simulink model "cyclo_mt"  (R2015b)
settings: Solver=FixedStepAuto  StartTime=0.0  StopTime=0.05  RelTol=1e-3
PreLoadFcn:
  | Ts=1e-6;
InitFcn:
  | DeadZone = 5;
  | block_angle = 90 - DeadZone;
  | Ts  = 1e-6;
  | fref = 50;
  | Eref = 400;
  | Em  = 4.16e3 * sqrt(2) / sqrt(3);
  | fao = 0;
undefined symbols (not defined in the file): D1, Delta, DiscIntNeverNeededParam, lagging, pulse
libraries: powerlib x26, powerlib_meascontrol x15, simulink x8
settings Model: Creator=fujitsu  LastModifiedBy=fujitsu

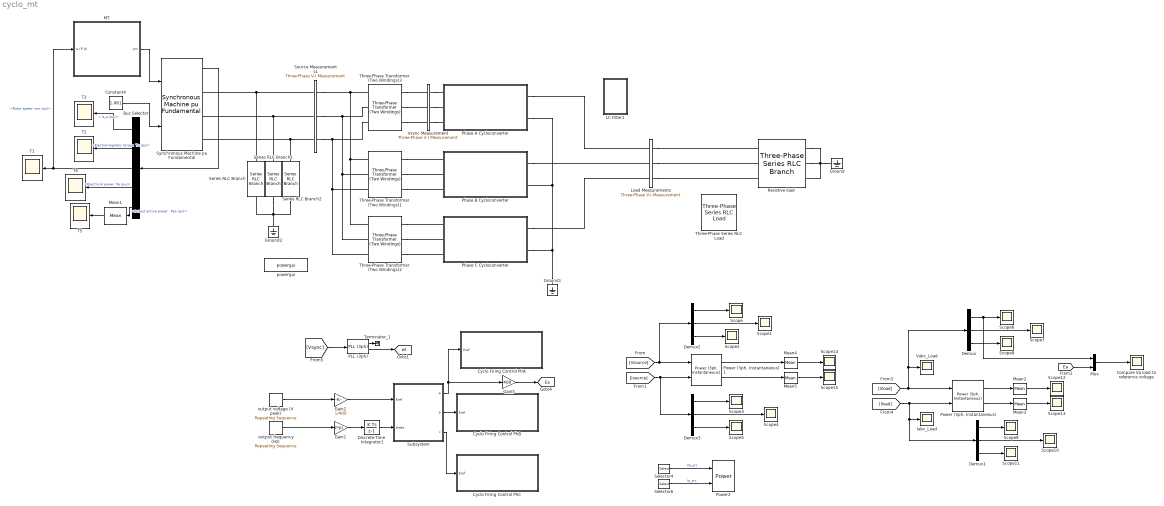
== system cyclo_mt ==
  Bus Selector : BusSelector  OutputSignals="Stator current. is_a (pu),Mechanical.Electromagnetic torque  Te (pu),Mechanical.Rotor speed  wm (pu),Mechanical.Electrical power  Pe (pu),Output active power   Peo (pu)"
  Compare Va load to reference voltage : Scope
  Constant4 : Constant  Value=1.061
  Cyclo Firing Control PhA : Subsystem
  Cyclo Firing Control PhB : Subsystem
  Cyclo Firing Control PhC : Subsystem
  Demux{,1..3} (4 alike) : Demux  Outputs=3
  Discrete-Time Integrator1 : DiscreteIntegrator  SampleTime=Ts  ICPrevOutput=DiscIntNeverNeededParam  ICPrevScaledInput=DiscIntNeverNeededParam
  Gain1 : Gain  Gain=2*pi
  Gain2 : Gain  Gain=1/400
  Gain5 : Gain  Gain=400
  Ground : powerlib/Elements/Ground  LConnTagsString=a
  Ground1 : powerlib/Elements/Ground  LConnTagsString=a
  Ground2 : powerlib/Elements/Ground  LConnTagsString=a
  Iabc_Load : Scope
  LC Filter1 : Subsystem
  Load Measurements : powerlib/Measurements/Three-Phase V-I Measurement  VoltageMeasurement=phase-to-ground  SetLabelV=on  LabelV=Vload  Vpu=off  VpuLL=off  CurrentMeasurement=yes  SetLabelI=on  LabelI=Iload  Ipu=off  Pbase=100e6  Vbase=500e3  OutputType=Complex  PhasorSimulation=off  PSBequivalent=0
  MT : Subsystem
  Mean{1..5} (5 alike) : powerlib_meascontrol/Measurements/Mean  Freq=50  Vinit=0  Ts=Ts
  Mux : Mux  Inputs=2
  PLL (3ph) : powerlib_meascontrol/PLL/PLL (3ph)  Fmin=45  Par_Init=[0, 50]  ParK=[180, 3200, 1]  TcD=1e-4  MaxRateChangeFreq=12  FilterCutOffFreq=25  Ts=Ts  AGC=on
  Phase A Cycloconverter : Subsystem
  Phase B Cycloconverter : Subsystem
  Phase C Cycloconverter : Subsystem
  "Power (3ph, Instantaneous)" : powerlib_meascontrol/Measurements/Power (3ph, Instantaneous)
  "Power (3ph, Instantaneous)1" : powerlib_meascontrol/Measurements/Power (3ph, Instantaneous)
  Power2 : powerlib_meascontrol/Measurements/Power  Freq=60  Vinit=[1, 0]  Iinit=[1, 0]  Ts=Ts
  Resistive load : powerlib/Elements/Three-Phase Series RLC Branch  LConnTagsString=A|B|C  RConnTagsString=A|B|C  BranchType=R  Resistance=100  Inductance=1e-3  Capacitance=1e-6  Measurements=None
  Scope{,1..15} (16 alike) : Scope
  Selector4 : Selector  InputPortWidth=3  IndexOptions=Index vector (dialog)  Indices=1  OutputSizes=1
  Selector6 : Selector  InputPortWidth=3  IndexOptions=Index vector (dialog)  Indices=1  OutputSizes=1
  Series RLC Branch : powerlib/Elements/Series RLC Branch  LConnTagsString=__new0  RConnTagsString=__new0  BranchType=C  Resistance=1  Inductance=1e-3  SetiL0=off  InitialCurrent=0  Capacitance=1e-9  Setx0=off  InitialVoltage=0  Measurements=None
  Series RLC Branch1 : powerlib/Elements/Series RLC Branch  LConnTagsString=__new0  RConnTagsString=__new0  BranchType=C  Resistance=1  Inductance=1e-3  SetiL0=off  InitialCurrent=0  Capacitance=1e-9  Setx0=off  InitialVoltage=0  Measurements=None
  Series RLC Branch2 : powerlib/Elements/Series RLC Branch  LConnTagsString=__new0  RConnTagsString=__new0  BranchType=C  Resistance=1  Inductance=1e-3  SetiL0=off  InitialCurrent=0  Capacitance=1e-9  Setx0=off  InitialVoltage=0  Measurements=None
  Source Measurements1 : powerlib/Measurements/Three-Phase V-I Measurement  VoltageMeasurement=phase-to-ground  SetLabelV=on  LabelV=Vsource  Vpu=off  VpuLL=off  CurrentMeasurement=yes  SetLabelI=on  LabelI=Isource  Ipu=off  Pbase=100e6  Vbase=500e3  OutputType=Complex  PhasorSimulation=off  PSBequivalent=0
  Subsystem : Subsystem
  Synchronous Machine pu Fundamental : powerlib/Machines/Synchronous Machine pu Fundamental  PresetModel=No  MechanicalLoad=Mechanical power Pm  ShowDetailedParameters=on  RotorType=Salient-pole  Units=per unit fundamental parameters  MeasurementBus=off  NominalParameters="[ 60e3  500 1500]"  Stator="[ 0.2503  0.114  0.6875  0.6875 ]"  Field="[ 1  10e15/(100*pi)]"  Dampers2=[0.0652, 0.5134, 0.0287, 0.2553, 7.765e-3, 0.9167 ]  Dampers1="[ 1.17E-02  0.182  1.97E-02  0.384 ]"  Mechanical=[ 6 0 2]  PolePairs=20  InitialConditions="[ 0  0  0  0  0  0  0  0  1 ]"  SetSaturation=off  Saturation=[0.6404,0.7127,0.8441,0.9214,0.9956,1.082,1.19,1.316,1.457;0.7,0.7698,0.8872,0.9466,0.9969,1.046,1.1,1.151,1.201]  LoadFlowParameters=[1,0,0,0,0]  TsPowergui=0  TsBlock=-1  IterativeModel=Trapezoidal non iterative  BusType=swing  Pref=0  Qref=0  Qmin=-inf  Qmax=inf  PLF=0  QLF=0
  T{1..5} (5 alike) : Scope
  Terminator_1 : Terminator
  Three-Phase Series RLC Load : powerlib/Elements/Three-Phase Series RLC Load  LConnTagsString=A|B|C  Configuration=Y (grounded)  NominalVoltage=400  Vabc=[1e3 1e3 1e3]  Vabcp=[1e3 1e3 1e3]  NominalFrequency=50  UnbalancedPower=off  ActivePower=10  InductivePower=0  CapacitivePower=0  Pabc=[10e3 9e3 11e3]  QLabc=[100 90 110]  QCabc=[100 90 110]  Pabcp=[10e3 9e3 11e3]  QLabcp=[100 90 110]  QCabcp=[100 90 110]  Measurements=None  LoadType=constant Z
  Three-Phase Transformer (Two Windings)1 : powerlib/Elements/Three-Phase Transformer (Two Windings)  Winding1Connection=Delta (D1)  Winding2Connection=Delta (D1)  CoreType=Three single-phase transformers  SetSaturation=off  Hysteresis=off  DataFile='hysteresis'  SetInitialFlux=off  Measurements=None  UNITS=pu  NominalPower=[3e6 1500]  Winding1=[500 0 0]  Winding2=[300 1e-8 0]  Rm=Inf  Lm=Inf  L0=0.5  Saturation=[ 0,0 ; 0.0024,1.2 ; 1.0,1.52 ]  InitialFluxes=[ 0.8 , -0.8 , 0.7 ]  MoreParameters=off  BreakLoop=off  DataType=off  TransfoNumber=1
  Three-Phase Transformer (Two Windings)2 : powerlib/Elements/Three-Phase Transformer (Two Windings)  Winding1Connection=Delta (D1)  Winding2Connection=Delta (D1)  CoreType=Three single-phase transformers  SetSaturation=off  Hysteresis=off  DataFile='hysteresis'  SetInitialFlux=off  Measurements=None  UNITS=pu  NominalPower=[3e6 1500]  Winding1=[500 0 0]  Winding2=[300 1e-8 0]  Rm=Inf  Lm=Inf  L0=0.5  Saturation=[ 0,0 ; 0.0024,1.2 ; 1.0,1.52 ]  InitialFluxes=[ 0.8 , -0.8 , 0.7 ]  MoreParameters=off  BreakLoop=off  DataType=off  TransfoNumber=1
  Three-Phase Transformer (Two Windings)3 : powerlib/Elements/Three-Phase Transformer (Two Windings)  Winding1Connection=Delta (D1)  Winding2Connection=Delta (D1)  CoreType=Three single-phase transformers  SetSaturation=off  Hysteresis=off  DataFile='hysteresis'  SetInitialFlux=off  Measurements=None  UNITS=pu  NominalPower=[3e6 1500]  Winding1=[500 0 0]  Winding2=[300 1e-8 0]  Rm=Inf  Lm=Inf  L0=0.5  Saturation=[ 0,0 ; 0.0024,1.2 ; 1.0,1.52 ]  InitialFluxes=[ 0.8 , -0.8 , 0.7 ]  MoreParameters=off  BreakLoop=off  DataType=off  TransfoNumber=1
  Vabc_Load : Scope
  Vsync Measurement : powerlib/Measurements/Three-Phase V-I Measurement  VoltageMeasurement=phase-to-ground  SetLabelV=on  LabelV=Vsync  Vpu=off  VpuLL=off  CurrentMeasurement=no  SetLabelI=off  LabelI=Iabc  Ipu=off  Pbase=100e6  Vbase=500e3  OutputType=Complex  PhasorSimulation=off  PSBequivalent=0
  output frequency (Hz) : simulink/Sources/Repeating Sequence  rep_seq_t=[0 10]  rep_seq_y=[1 1]*50
  output voltage (V peak) : simulink/Sources/Repeating Sequence  rep_seq_t=[0 10]  rep_seq_y=[1 1]*400
  powergui : powerlib/powergui  SimulationMode=Discrete  SolverType=Backward Euler  SampleTime=Ts  frequency=60  SPID=off  DisableSnubberDevices=off  DisableRonSwitches=off  DisableVfSwitches=off  SwTol=0  DisplayEquations=off  Interpol=off  ExternalGateDelay=off  methode=off  Ts=0  FunctionMessages=off  echomessages=off  HookPort=off  EnableUseOfTLC=off  x0status=blocks  frequencyindice=0  Pbase=100e6  ErrMax=1e-4  Iterations=50  UnitsV=kV  UnitsW=MW  buscounter=0  RestoreLinks=warning  ResistiveCurrentMeasurement=off  Frange=[0:2:500]  Ylog=off  Xlog=on  ShowGrid=off  save=off  variable=ZData  structure=VaLoad  ZoomFFT=off  StartTime=0.3  cycles=1  DisplayStyle=2  fundamental=10  FreqAxis=on  MaxFrequency=500  frequencyindicesteady=1  RmsSteady=1  display=off
  tag scope: Ea=global, wt=global
  wires:
  MT/1(pm) -> Synchronous Machine pu Fundamental/1
  Synchronous Machine pu Fundamental/1 -> Bus Selector/1
  Bus Selector/1 -> T3/1  "< is_a (pu)>"
  Bus Selector/2 -> T2/1  "<Electromagnetic torque  Te (pu)>"
  Bus Selector/3 -> MT/1(w (P.U)), T1/1  "<Rotor speed  wm (pu)>"
  Constant4/1 -> Synchronous Machine pu Fundamental/2
  Bus Selector/4 -> T4/1  "<Electrical power  Pe (pu)>"
  Bus Selector/5 -> Mean1/1  "<Output active power   Peo (pu)>"
  Mean1/1 -> T5/1
  Mux/1 -> Compare Va load to reference voltage/1
  [Ea] -> Mux/2
  [Vsource] -> "Power (3ph, Instantaneous)1"/1, Demux2/1
  [Iload] -> Demux1/1, Iabc_Load/1, "Power (3ph, Instantaneous)"/2
  [Vload] -> Demux/1, Vabc_Load/1, "Power (3ph, Instantaneous)"/1
  [Isource] -> Demux3/1, "Power (3ph, Instantaneous)1"/2
  Demux2/1 -> Scope/1
  Demux2/2 -> Scope1/1
  Demux2/3 -> Scope2/1
  Demux3/1 -> Scope3/1
  Demux3/2 -> Scope4/1
  Demux3/3 -> Scope5/1
  Demux/1 -> Mux/1, Scope6/1
  Demux/2 -> Scope7/1
  Demux/3 -> Scope8/1
  Demux1/1 -> Scope9/1
  Demux1/2 -> Scope10/1
  Demux1/3 -> Scope11/1
  Mean2/1 -> Scope12/1
  Mean3/1 -> Scope13/1
  Mean4/1 -> Scope14/1
  Mean5/1 -> Scope15/1
  Selector4/1 -> Power2/1  "Va_src"
  Selector6/1 -> Power2/2  "Ia_src"
  "Power (3ph, Instantaneous)"/1 -> Mean2/1
  "Power (3ph, Instantaneous)"/2 -> Mean3/1
  "Power (3ph, Instantaneous)1"/1 -> Mean4/1
  "Power (3ph, Instantaneous)1"/2 -> Mean5/1
  Discrete-Time Integrator1/1 -> Subsystem/2(theta)
  Subsystem/2(b) -> Cyclo Firing Control PhB/1(Eref)
  Subsystem/1(a) -> Cyclo Firing Control PhA/1(Eref), Gain5/1
  Subsystem/3(c) -> Cyclo Firing Control PhC/1(Eref)
  output frequency (Hz)/1 -> Gain1/1
  Gain1/1 -> Discrete-Time Integrator1/1
  Gain5/1 -> [Ea]
  output voltage (V peak)/1 -> Gain2/1
  Gain2/1 -> Subsystem/1(Eref)
  [Vsync] -> PLL (3ph)/1
  PLL (3ph)/2 -> [wt]
  PLL (3ph)/1 -> Terminator_1/1
  connections:
  Ground/LConn1 -- Resistive load/RConn2 -- Resistive load/RConn1 -- Resistive load/RConn3
  Ground1/LConn1 -- Phase C Cycloconverter/RConn2 -- Phase A Cycloconverter/RConn2 -- Phase B Cycloconverter/RConn2
  Vsync Measurement/RConn1 -- Phase A Cycloconverter/LConn1
  Vsync Measurement/RConn2 -- Phase A Cycloconverter/LConn2
  Vsync Measurement/RConn3 -- Phase A Cycloconverter/LConn3
  Three-Phase Transformer (Two Windings)3/LConn1 -- Source Measurements1/RConn1 -- Three-Phase Transformer (Two Windings)2/LConn1 -- Three-Phase Transformer (Two Windings)1/LConn1
  Three-Phase Transformer (Two Windings)3/LConn2 -- Source Measurements1/RConn2 -- Three-Phase Transformer (Two Windings)2/LConn2 -- Three-Phase Transformer (Two Windings)1/LConn2
  Three-Phase Transformer (Two Windings)3/LConn3 -- Source Measurements1/RConn3 -- Three-Phase Transformer (Two Windings)2/LConn3 -- Three-Phase Transformer (Two Windings)1/LConn3
  Ground2/LConn1 -- Series RLC Branch2/RConn1 -- Series RLC Branch1/RConn1 -- Series RLC Branch/RConn1
  Three-Phase Transformer (Two Windings)3/RConn1 -- Vsync Measurement/LConn1
  Three-Phase Transformer (Two Windings)3/RConn2 -- Vsync Measurement/LConn2
  Three-Phase Transformer (Two Windings)3/RConn3 -- Vsync Measurement/LConn3
  Three-Phase Transformer (Two Windings)1/RConn1 -- Phase B Cycloconverter/LConn1
  Three-Phase Transformer (Two Windings)1/RConn2 -- Phase B Cycloconverter/LConn2
  Three-Phase Transformer (Two Windings)1/RConn3 -- Phase B Cycloconverter/LConn3
  Three-Phase Transformer (Two Windings)2/RConn1 -- Phase C Cycloconverter/LConn1
  Three-Phase Transformer (Two Windings)2/RConn2 -- Phase C Cycloconverter/LConn2
  Three-Phase Transformer (Two Windings)2/RConn3 -- Phase C Cycloconverter/LConn3
  Phase C Cycloconverter/RConn1 -- Load Measurements/LConn3
  Phase B Cycloconverter/RConn1 -- Load Measurements/LConn2
  Phase A Cycloconverter/RConn1 -- Load Measurements/LConn1
  Source Measurements1/LConn2 -- Series RLC Branch1/LConn1 -- Synchronous Machine pu Fundamental/RConn2
  Source Measurements1/LConn3 -- Series RLC Branch2/LConn1 -- Synchronous Machine pu Fundamental/RConn3
  Series RLC Branch/LConn1 -- Synchronous Machine pu Fundamental/RConn1 -- Source Measurements1/LConn1
  Load Measurements/RConn1 -- Resistive load/LConn1
  Load Measurements/RConn2 -- Resistive load/LConn2
  Load Measurements/RConn3 -- Resistive load/LConn3

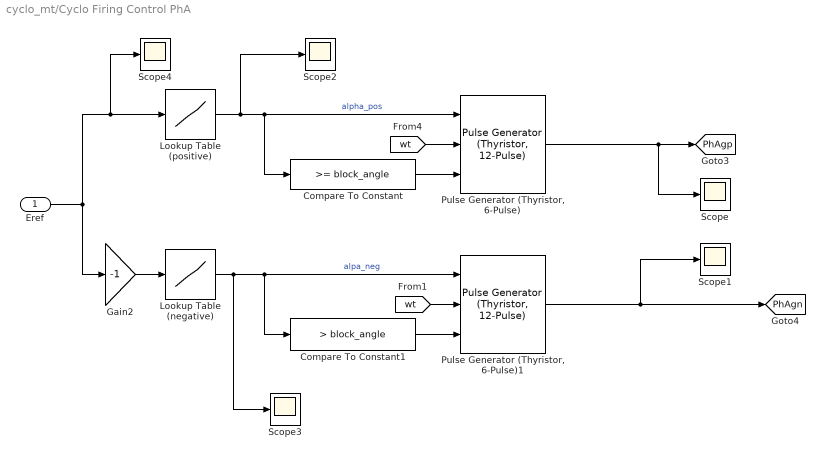
== system cyclo_mt/Cyclo Firing Control PhA ==
  Eref : Inport
  Compare To Constant : simulink/Logic and Bit Operations/Compare To Constant  relop=>=  const=block_angle  OutDataTypeStr=boolean  ZeroCross=off
  Compare To Constant1 : simulink/Logic and Bit Operations/Compare To Constant  relop=>  const=block_angle  OutDataTypeStr=boolean  ZeroCross=off
  Gain2 : Gain  Gain=-1
  Lookup Table (negative) : Lookup  InputValues=[-1 0 1]  Table=[90 90 0]+fao
  Lookup Table (positive) : Lookup  InputValues=[-1 0 1]  Table=[90 90 0]+fao
  "Pulse Generator (Thyristor, 6-Pulse)" : powerlib_meascontrol/Pulse & Signal Generators/Pulse Generator (Thyristor, 12-Pulse)  GenType=6-pulse  Delta=D1 (lagging)  pwidth=150  Double_Pulse=off  Ts=Ts
  "Pulse Generator (Thyristor, 6-Pulse)1" : powerlib_meascontrol/Pulse & Signal Generators/Pulse Generator (Thyristor, 12-Pulse)  GenType=6-pulse  Delta=D1 (lagging)  pwidth=150  Double_Pulse=off  Ts=Ts
  Scope{,1..4} (5 alike) : Scope
  tag scope: PhAgn=global, PhAgp=global
  wires:
  "Pulse Generator (Thyristor, 6-Pulse)"/1 -> Scope/1, [PhAgp]
  "Pulse Generator (Thyristor, 6-Pulse)1"/1 -> Scope1/1, [PhAgn]
  Compare To Constant/1 -> "Pulse Generator (Thyristor, 6-Pulse)"/3
  Lookup Table (positive)/1 -> Scope2/1, "Pulse Generator (Thyristor, 6-Pulse)"/1, Compare To Constant/1  "alpha_pos"
  Lookup Table (negative)/1 -> Scope3/1, Compare To Constant1/1, "Pulse Generator (Thyristor, 6-Pulse)1"/1  "alpa_neg"
  Eref/1 -> Scope4/1, Lookup Table (positive)/1, Gain2/1
  Compare To Constant1/1 -> "Pulse Generator (Thyristor, 6-Pulse)1"/3
  Gain2/1 -> Lookup Table (negative)/1
  [wt] -> "Pulse Generator (Thyristor, 6-Pulse)"/2
  [wt] -> "Pulse Generator (Thyristor, 6-Pulse)1"/2

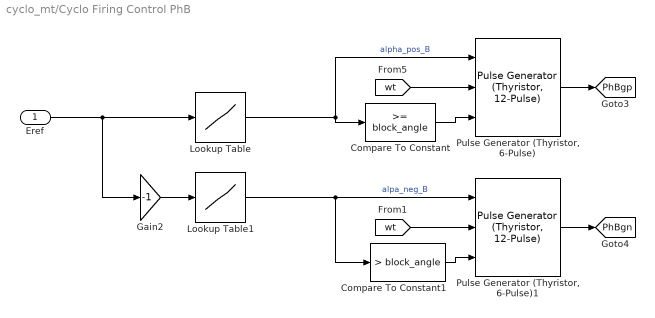
== system cyclo_mt/Cyclo Firing Control PhB ==
  Eref : Inport
  Compare To Constant : simulink/Logic and Bit Operations/Compare To Constant  relop=>=  const=block_angle  OutDataTypeStr=boolean  ZeroCross=off
  Compare To Constant1 : simulink/Logic and Bit Operations/Compare To Constant  relop=>  const=block_angle  OutDataTypeStr=boolean  ZeroCross=off
  Gain2 : Gain  Gain=-1
  Lookup Table : Lookup  InputValues=[-1 0 1]  Table=[90 90 0]+fao
  Lookup Table1 : Lookup  InputValues=[-1 0 1]  Table=[90 90 0]+fao
  "Pulse Generator (Thyristor, 6-Pulse)" : powerlib_meascontrol/Pulse & Signal Generators/Pulse Generator (Thyristor, 12-Pulse)  GenType=6-pulse  Delta=D1 (lagging)  pwidth=150  Double_Pulse=off  Ts=Ts
  "Pulse Generator (Thyristor, 6-Pulse)1" : powerlib_meascontrol/Pulse & Signal Generators/Pulse Generator (Thyristor, 12-Pulse)  GenType=6-pulse  Delta=D1 (lagging)  pwidth=150  Double_Pulse=off  Ts=Ts
  tag scope: PhBgn=global, PhBgp=global
  wires:
  Eref/1 -> Lookup Table/1, Gain2/1
  Lookup Table1/1 -> "Pulse Generator (Thyristor, 6-Pulse)1"/1, Compare To Constant1/1  "alpa_neg_B"
  Lookup Table/1 -> Compare To Constant/1, "Pulse Generator (Thyristor, 6-Pulse)"/1  "alpha_pos_B"
  Compare To Constant/1 -> "Pulse Generator (Thyristor, 6-Pulse)"/3
  [wt] -> "Pulse Generator (Thyristor, 6-Pulse)"/2
  "Pulse Generator (Thyristor, 6-Pulse)1"/1 -> [PhBgn]
  "Pulse Generator (Thyristor, 6-Pulse)"/1 -> [PhBgp]
  Compare To Constant1/1 -> "Pulse Generator (Thyristor, 6-Pulse)1"/3
  Gain2/1 -> Lookup Table1/1
  [wt] -> "Pulse Generator (Thyristor, 6-Pulse)1"/2

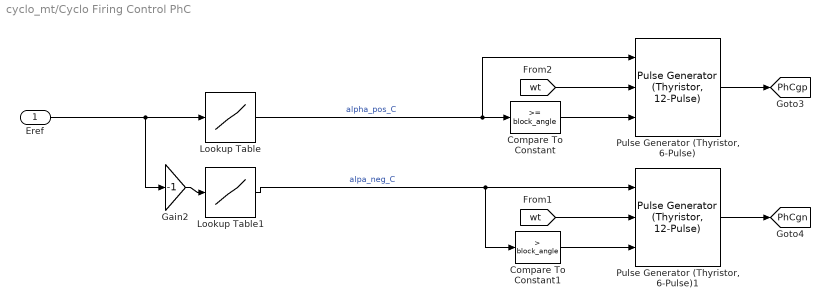
== system cyclo_mt/Cyclo Firing Control PhC ==
  Eref : Inport
  Compare To Constant : simulink/Logic and Bit Operations/Compare To Constant  relop=>=  const=block_angle  OutDataTypeStr=boolean  ZeroCross=off
  Compare To Constant1 : simulink/Logic and Bit Operations/Compare To Constant  relop=>  const=block_angle  OutDataTypeStr=boolean  ZeroCross=off
  Gain2 : Gain  Gain=-1
  Lookup Table : Lookup  InputValues=[-1 0 1]  Table=[90 90 0]+fao
  Lookup Table1 : Lookup  InputValues=[-1 0 1]  Table=[90 90 0]+fao
  "Pulse Generator (Thyristor, 6-Pulse)" : powerlib_meascontrol/Pulse & Signal Generators/Pulse Generator (Thyristor, 12-Pulse)  GenType=6-pulse  Delta=D1 (lagging)  pwidth=120  Double_Pulse=off  Ts=Ts
  "Pulse Generator (Thyristor, 6-Pulse)1" : powerlib_meascontrol/Pulse & Signal Generators/Pulse Generator (Thyristor, 12-Pulse)  GenType=6-pulse  Delta=D1 (lagging)  pwidth=120  Double_Pulse=off  Ts=Ts
  tag scope: PhCgn=global, PhCgp=global
  wires:
  "Pulse Generator (Thyristor, 6-Pulse)"/1 -> [PhCgp]
  "Pulse Generator (Thyristor, 6-Pulse)1"/1 -> [PhCgn]
  Lookup Table/1 -> "Pulse Generator (Thyristor, 6-Pulse)"/1, Compare To Constant/1  "alpha_pos_C"
  Lookup Table1/1 -> Compare To Constant1/1, "Pulse Generator (Thyristor, 6-Pulse)1"/1  "alpa_neg_C"
  Eref/1 -> Lookup Table/1, Gain2/1
  Compare To Constant1/1 -> "Pulse Generator (Thyristor, 6-Pulse)1"/3
  Gain2/1 -> Lookup Table1/1
  [wt] -> "Pulse Generator (Thyristor, 6-Pulse)1"/2
  Compare To Constant/1 -> "Pulse Generator (Thyristor, 6-Pulse)"/3
  [wt] -> "Pulse Generator (Thyristor, 6-Pulse)"/2

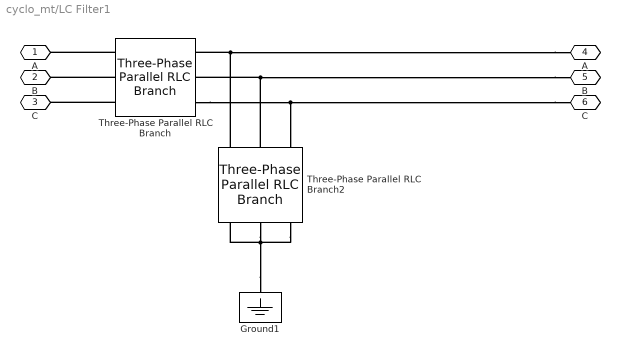
== system cyclo_mt/LC Filter1 ==
  Ground1 : powerlib/Elements/Ground  LConnTagsString=a
  Three-Phase Parallel RLC Branch : powerlib/Elements/Three-Phase Parallel RLC Branch  LConnTagsString=A|B|C  RConnTagsString=A|B|C  BranchType=L  Resistance=1  Inductance=6e-3  Capacitance=1e-6  Measurements=None
  Three-Phase Parallel RLC Branch2 : powerlib/Elements/Three-Phase Parallel RLC Branch  LConnTagsString=A|B|C  RConnTagsString=A|B|C  BranchType=C  Resistance=1  Inductance=5.7e-3  Capacitance=1000e-6  Measurements=None
  A : PMIOPort  Port=1  Side=Left
  B : PMIOPort  Port=2  Side=Left
  C : PMIOPort  Port=3  Side=Left
  "A " : PMIOPort  Port=4  Side=Right
  "B " : PMIOPort  Port=5  Side=Right
  "C " : PMIOPort  Port=6  Side=Right
  connections:
  Ground1/LConn1 -- Three-Phase Parallel RLC Branch2/RConn3 -- Three-Phase Parallel RLC Branch2/RConn1 -- Three-Phase Parallel RLC Branch2/RConn2
  Three-Phase Parallel RLC Branch/LConn3 -- C/RConn1
  Three-Phase Parallel RLC Branch/LConn2 -- B/RConn1
  Three-Phase Parallel RLC Branch/LConn1 -- A/RConn1
  "A "/RConn1 -- Three-Phase Parallel RLC Branch/RConn1 -- Three-Phase Parallel RLC Branch2/LConn1
  "B "/RConn1 -- Three-Phase Parallel RLC Branch/RConn2 -- Three-Phase Parallel RLC Branch2/LConn2
  "C "/RConn1 -- Three-Phase Parallel RLC Branch2/LConn3 -- Three-Phase Parallel RLC Branch/RConn3

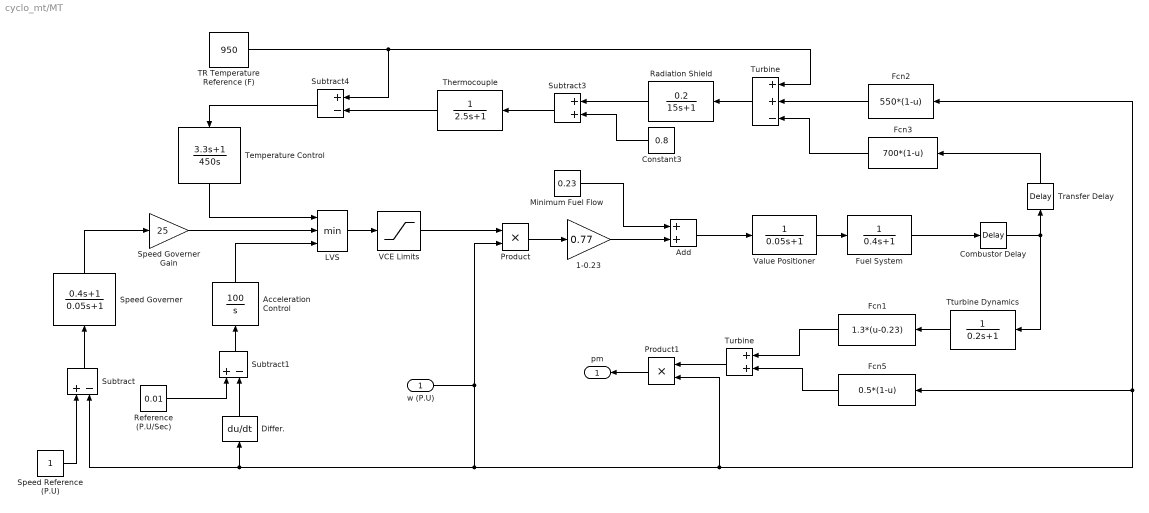
== system cyclo_mt/MT ==
  w (P.U) : Inport
  1-0.23 : Gain  Gain=0.77
  Acceleration Control : TransferFcn  Numerator=[0 100]  Denominator=[1 0]
  Add : Sum
  Combustor Delay : TransportDelay  DelayTime=0.01
  Constant3 : Constant  Value=0.8
  Differ. : Derivative
  Fcn1 : Fcn  Expr=1.3*(u-0.23)
  Fcn2 : Fcn  Expr=550*(1-u)
  Fcn3 : Fcn  Expr=700*(1-u)
  Fcn5 : Fcn  Expr=0.5*(1-u)
  Fuel System : TransferFcn  Denominator=[0.4 1]
  LVS : MinMax  Inputs=3
  Minimum Fuel Flow : Constant  Value=0.23
  Product : Product  RndMeth=Zero
  Product1 : Product  RndMeth=Zero
  Radiation Shield : TransferFcn  Numerator=[0.2]  Denominator=[15 1]
  Reference (P.U/Sec) : Constant  Value=0.01
  Speed Governer : TransferFcn  Numerator=[0.4 1]  Denominator=[0.05 1]
  Speed Governer Gain : Gain  Gain=25
  Speed Reference (P.U) : Constant
  Subtract : Sum  Inputs=+-
  Subtract1 : Sum  Inputs=+-
  Subtract3 : Sum
  Subtract4 : Sum  Inputs=+-
  TR Temperature Reference (F) : Constant  Value=950
  Temperature Control : TransferFcn  Numerator=[3.3 1]  Denominator=[450 0]
  Thermocouple : TransferFcn  Denominator=[2.5 1]
  Transfer Delay : TransportDelay  DelayTime=0.04
  Tturbine Dynamics : TransferFcn  Denominator=[0.2 1]
  Turbine : Sum  Inputs=++-
  "Turbine " : Sum
  VCE Limits : Saturate  UpperLimit=1.5  LowerLimit=-0.1
  Value Positioner : TransferFcn  Denominator=[0.05 1]
  pm : Outport
  wires:
  Speed Reference (P.U)/1 -> Subtract/1
  Subtract/1 -> Speed Governer/1
  VCE Limits/1 -> Product/1
  Product/1 -> 1-0.23/1
  1-0.23/1 -> Add/2
  Minimum Fuel Flow/1 -> Add/1
  Add/1 -> Value Positioner/1
  Value Positioner/1 -> Fuel System/1
  Fuel System/1 -> Combustor Delay/1
  Combustor Delay/1 -> Tturbine Dynamics/1, Transfer Delay/1
  Speed Governer Gain/1 -> LVS/2
  Differ./1 -> Subtract1/2
  Reference (P.U/Sec)/1 -> Subtract1/1
  Subtract1/1 -> Acceleration Control/1
  Acceleration Control/1 -> LVS/3
  LVS/1 -> VCE Limits/1
  Transfer Delay/1 -> Fcn3/1
  Fcn3/1 -> Turbine/3
  Fcn2/1 -> Turbine/2
  Radiation Shield/1 -> Subtract3/1
  Constant3/1 -> Subtract3/2
  Turbine/1 -> Radiation Shield/1
  Subtract3/1 -> Thermocouple/1
  Thermocouple/1 -> Subtract4/2
  TR Temperature Reference (F)/1 -> Turbine/1, Subtract4/1
  Subtract4/1 -> Temperature Control/1
  Temperature Control/1 -> LVS/1
  Speed Governer/1 -> Speed Governer Gain/1
  w (P.U)/1 -> Product/2, Subtract/2, Differ./1, Product1/2, Fcn5/1, Fcn2/1
  Tturbine Dynamics/1 -> Fcn1/1
  Fcn1/1 -> "Turbine "/1
  Fcn5/1 -> "Turbine "/2
  "Turbine "/1 -> Product1/1
  Product1/1 -> pm/1

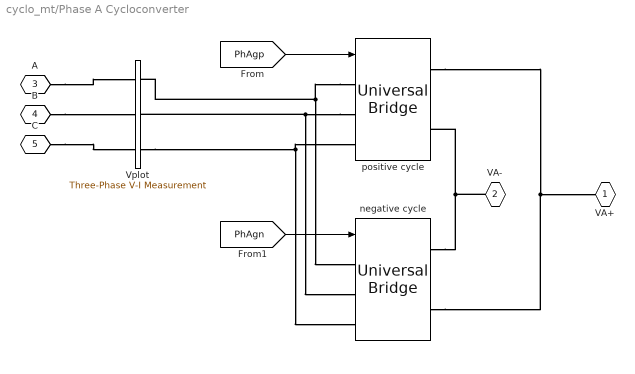
== system cyclo_mt/Phase A Cycloconverter ==
  Vplot : powerlib/Measurements/Three-Phase V-I Measurement  VoltageMeasurement=no  SetLabelV=off  LabelV=Vplot  Vpu=off  VpuLL=off  CurrentMeasurement=no  SetLabelI=off  LabelI=Iabc  Ipu=off  Pbase=100e6  Vbase=500e3  OutputType=Complex  PhasorSimulation=off  PSBequivalent=0
  negative cycle : powerlib/Power Electronics/Universal Bridge  Arms=3  SnubberResistance=1e3  SnubberCapacitance=1e-7  Device=Thyristors  Ron=1e-5  Lon=0  ForwardVoltages="[  0  0  ]"  ForwardVoltage=0  GTOparameters=[ 10e-6 , 20e-6 ]  IGBTparameters=[ 1e-6 , 2e-6 ]  Measurements=None  Measurements_2=None  converterType=Rectifier
  positive cycle : powerlib/Power Electronics/Universal Bridge  Arms=3  SnubberResistance=1e3  SnubberCapacitance=1e-7  Device=Thyristors  Ron=1e-5  Lon=0  ForwardVoltages="[  0  0  ]"  ForwardVoltage=0  GTOparameters=[ 10e-6 , 20e-6 ]  IGBTparameters=[ 1e-6 , 2e-6 ]  Measurements=None  Measurements_2=None  converterType=Rectifier
  VA+ : PMIOPort  Tag=PMCPort  Port=1  Side=Right
  VA- : PMIOPort  Tag=PMCPort  Port=2  Side=Right
  A : PMIOPort  Tag=PMCPort  Port=3  Side=Left
  B : PMIOPort  Tag=PMCPort  Port=4  Side=Left
  C : PMIOPort  Tag=PMCPort  Port=5  Side=Left
  wires:
  [PhAgp] -> positive cycle/1
  [PhAgn] -> negative cycle/1
  connections:
  positive cycle/LConn1 -- negative cycle/LConn1 -- Vplot/RConn1
  positive cycle/LConn2 -- Vplot/RConn2 -- negative cycle/LConn2
  Vplot/RConn3 -- positive cycle/LConn3 -- negative cycle/LConn3
  negative cycle/RConn1 -- positive cycle/RConn2 -- VA-/RConn1
  positive cycle/RConn1 -- VA+/RConn1 -- negative cycle/RConn2
  B/RConn1 -- Vplot/LConn2
  C/RConn1 -- Vplot/LConn3
  A/RConn1 -- Vplot/LConn1

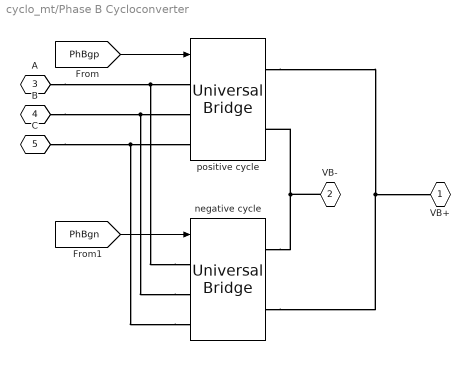
== system cyclo_mt/Phase B Cycloconverter ==
  negative cycle : powerlib/Power Electronics/Universal Bridge  Arms=3  SnubberResistance=1e3  SnubberCapacitance=1e-7  Device=Thyristors  Ron=1e-5  Lon=0  ForwardVoltages="[  0  0  ]"  ForwardVoltage=0  GTOparameters=[ 10e-6 , 20e-6 ]  IGBTparameters=[ 1e-6 , 2e-6 ]  Measurements=None  Measurements_2=None  converterType=Rectifier
  positive cycle : powerlib/Power Electronics/Universal Bridge  Arms=3  SnubberResistance=1e3  SnubberCapacitance=1e-7  Device=Thyristors  Ron=1e-5  Lon=0  ForwardVoltages="[  0  0  ]"  ForwardVoltage=0  GTOparameters=[ 10e-6 , 20e-6 ]  IGBTparameters=[ 1e-6 , 2e-6 ]  Measurements=None  Measurements_2=None  converterType=Rectifier
  VB+ : PMIOPort  Tag=PMCPort  Port=1  Side=Right
  VB- : PMIOPort  Tag=PMCPort  Port=2  Side=Right
  A : PMIOPort  Tag=PMCPort  Port=3  Side=Left
  B : PMIOPort  Tag=PMCPort  Port=4  Side=Left
  C : PMIOPort  Tag=PMCPort  Port=5  Side=Left
  wires:
  [PhBgn] -> negative cycle/1
  [PhBgp] -> positive cycle/1
  connections:
  negative cycle/RConn2 -- VB+/RConn1 -- positive cycle/RConn1
  VB-/RConn1 -- positive cycle/RConn2 -- negative cycle/RConn1
  negative cycle/LConn3 -- positive cycle/LConn3 -- C/RConn1
  negative cycle/LConn2 -- positive cycle/LConn2 -- B/RConn1
  negative cycle/LConn1 -- positive cycle/LConn1 -- A/RConn1

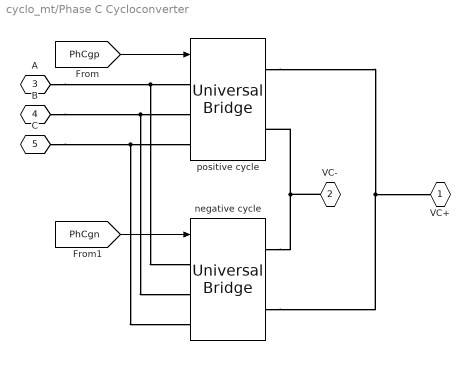
== system cyclo_mt/Phase C Cycloconverter ==
  negative cycle : powerlib/Power Electronics/Universal Bridge  Arms=3  SnubberResistance=1e3  SnubberCapacitance=1e-7  Device=Thyristors  Ron=1e-5  Lon=0  ForwardVoltages="[  0  0  ]"  ForwardVoltage=0  GTOparameters=[ 10e-6 , 20e-6 ]  IGBTparameters=[ 1e-6 , 2e-6 ]  Measurements=None  Measurements_2=None  converterType=Rectifier
  positive cycle : powerlib/Power Electronics/Universal Bridge  Arms=3  SnubberResistance=1e3  SnubberCapacitance=1e-7  Device=Thyristors  Ron=1e-5  Lon=0  ForwardVoltages="[  0  0  ]"  ForwardVoltage=0  GTOparameters=[ 10e-6 , 20e-6 ]  IGBTparameters=[ 1e-6 , 2e-6 ]  Measurements=None  Measurements_2=None  converterType=Rectifier
  VC+ : PMIOPort  Tag=PMCPort  Port=1  Side=Right
  VC- : PMIOPort  Tag=PMCPort  Port=2  Side=Right
  A : PMIOPort  Tag=PMCPort  Port=3  Side=Left
  B : PMIOPort  Tag=PMCPort  Port=4  Side=Left
  C : PMIOPort  Tag=PMCPort  Port=5  Side=Left
  wires:
  [PhCgp] -> positive cycle/1
  [PhCgn] -> negative cycle/1
  connections:
  A/RConn1 -- positive cycle/LConn1 -- negative cycle/LConn1
  B/RConn1 -- positive cycle/LConn2 -- negative cycle/LConn2
  C/RConn1 -- positive cycle/LConn3 -- negative cycle/LConn3
  negative cycle/RConn1 -- positive cycle/RConn2 -- VC-/RConn1
  positive cycle/RConn1 -- VC+/RConn1 -- negative cycle/RConn2

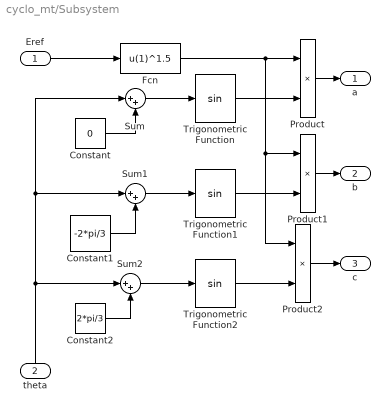
== system cyclo_mt/Subsystem ==
  Eref : Inport
  theta : Inport  Port=2
  Constant : Constant  Value=0
  Constant1 : Constant  Value=-2*pi/3
  Constant2 : Constant  Value=2*pi/3
  Fcn : Fcn  Expr=u(1)^1.5
  Product : Product  RndMeth=Zero
  Product1 : Product  RndMeth=Zero
  Product2 : Product  RndMeth=Zero
  Sum : Sum  Inputs=|++
  Sum1 : Sum  Inputs=|++
  Sum2 : Sum  Inputs=|++
  Trigonometric Function : Trigonometry
  Trigonometric Function1 : Trigonometry
  Trigonometric Function2 : Trigonometry
  a : Outport
  b : Outport  Port=2
  c : Outport  Port=3
  wires:
  theta/1 -> Sum1/1, Sum/1, Sum2/1
  Sum/1 -> Trigonometric Function/1
  Constant/1 -> Sum/2
  Trigonometric Function/1 -> Product/2
  Sum1/1 -> Trigonometric Function1/1
  Constant1/1 -> Sum1/2
  Trigonometric Function1/1 -> Product1/2
  Sum2/1 -> Trigonometric Function2/1
  Constant2/1 -> Sum2/2
  Trigonometric Function2/1 -> Product2/2
  Eref/1 -> Fcn/1
  Product/1 -> a/1
  Product1/1 -> b/1
  Product2/1 -> c/1
  Fcn/1 -> Product/1, Product1/1, Product2/1
